simulink model "kalmanHung"  (R2016a)
settings: Solver=VariableStepAuto  StartTime=0.0  StopTime=10  RelTol=1e-3
libraries: commrandsrc3 x1
settings Model: Creator=hung  LastModifiedBy=hung

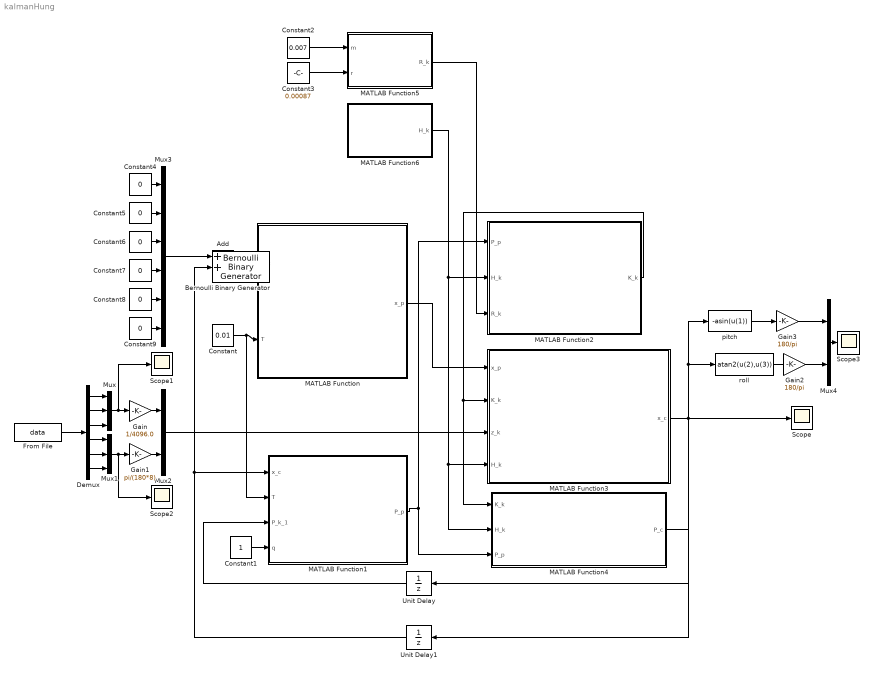
== system kalmanHung ==
  Add : Sum
  Constant : Constant  Value=0.01
  Constant1 : Constant
  Constant2 : Constant  Value=0.007
  Constant3 : Constant  Value=0.00087
  Constant{4..9} (6 alike) : Constant  Value=0
  Demux : Demux  Outputs=6
  From File : FromFile  FileName=data  SampleTime=0.01
  Gain : Gain  Gain=1/4096.0
  Gain1 : Gain  Gain=pi/(180*8)
  Gain2 : Gain  Gain=180/pi
  Gain3 : Gain  Gain=180/pi
  MATLAB Function : MATLAB Function  InitFcn=x_c=[0 0 0 0 0 0 ]'  TreatAsAtomicUnit=on
  MATLAB Function1 : MATLAB Function  TreatAsAtomicUnit=on
  MATLAB Function2 : MATLAB Function  TreatAsAtomicUnit=on
  MATLAB Function3 : MATLAB Function  TreatAsAtomicUnit=on
  MATLAB Function4 : MATLAB Function  TreatAsAtomicUnit=on
  MATLAB Function5 : MATLAB Function  TreatAsAtomicUnit=on
  MATLAB Function6 : MATLAB Function  TreatAsAtomicUnit=on
  Mux : Mux  Inputs=3
  Mux1 : Mux  Inputs=3
  Mux2 : Mux  Inputs=2
  Mux3 : Mux  Inputs=6
  Mux4 : Mux  Inputs=2
  Scope{,1..3} (4 alike) : Scope
  Unit Delay : UnitDelay  InitialCondition=eye(6,6)  SampleTime=-1
  Unit Delay1 : UnitDelay  InitialCondition=zeros(6,1)  SampleTime=-1
  pitch : Fcn  Expr=-asin(u(1))
  roll : Fcn  Expr=atan2(u(2),u(3))
  Bernoulli Binary Generator : commrandsrc3/Bernoulli Binary Generator  IOType=siggen  ProbabilityOfZero=0.5  SeedSource=Auto  Seed=0  SampleTime=1  SamplesPerFrame=1  OutputDataType=double  SimulateUsing=Interpreted execution
  wires:
  MATLAB Function/1(x_p) -> MATLAB Function3/1(x_p)
  MATLAB Function1/1(P_p) -> MATLAB Function4/3(P_p), MATLAB Function2/1(P_p)
  MATLAB Function2/1(K_k) -> MATLAB Function4/1(K_k), MATLAB Function3/2(K_k)
  MATLAB Function4/1(P_c) -> Unit Delay/1
  Constant1/1 -> MATLAB Function1/4(q)
  Constant/1 -> MATLAB Function1/2(T), MATLAB Function/2(T)
  MATLAB Function5/1(R_k) -> MATLAB Function2/3(R_k)
  MATLAB Function6/1(H_k) -> MATLAB Function3/4(H_k), MATLAB Function4/2(H_k), MATLAB Function2/2(H_k)
  Constant2/1 -> MATLAB Function5/1(m)
  Constant3/1 -> MATLAB Function5/2(r)
  From File/1 -> Demux/1
  Demux/1 -> Mux/1
  Demux/2 -> Mux/2
  Demux/3 -> Mux/3
  Demux/4 -> Mux1/1
  Demux/5 -> Mux1/2
  Demux/6 -> Mux1/3
  Mux/1 -> Scope1/1, Gain/1
  Mux1/1 -> Scope2/1, Gain1/1
  Gain/1 -> Mux2/1
  Gain1/1 -> Mux2/2
  Mux2/1 -> MATLAB Function3/3(z_k)
  Add/1 -> MATLAB Function/1(x_c)
  Mux3/1 -> Add/1
  Constant4/1 -> Mux3/1
  Constant5/1 -> Mux3/2
  Constant6/1 -> Mux3/3
  Constant7/1 -> Mux3/4
  Constant8/1 -> Mux3/5
  Constant9/1 -> Mux3/6
  Unit Delay/1 -> MATLAB Function1/3(P_k_1)
  Unit Delay1/1 -> Add/2, MATLAB Function1/1(x_c)
  MATLAB Function3/1(x_c) -> Scope/1, Unit Delay1/1, roll/1, pitch/1
  roll/1 -> Mux4/2
  pitch/1 -> Gain3/1
  Mux4/1 -> Scope3/1
  Gain3/1 -> Mux4/1

== matlab function kalmanHung/MATLAB Function1 ==
  data: x_c input; P_p output; T input; P_k_1 input; q input
function P_p=Predict_P(x_c,T,P_k_1,q)% x_p: x predicted, x_c: x_corrected
C3=[0,-x_c(3),x_c(2);x_c(3),0,-x_c(1);-x_c(2),x_c(1),0];
Ak=[eye(3,3),T*C3;zeros(3,3),eye(3,3)];
Qk=q*[T^3*C3*C3',T^2*C3;T^2*C3',T*eye(3,3)];
P_p=Ak*P_k_1*Ak'+Qk;
end

== matlab function kalmanHung/MATLAB Function ==
  data: x_c input; x_p output; T input
function x_p=Predict_x(x_c,T)% x_p: x predicted, x_c: x_corrected
C3=[0,-x_c(3),x_c(2);x_c(3),0,-x_c(1);-x_c(2),x_c(1),0];
Ak=[eye(3,3),T*C3;zeros(3,3),eye(3,3)];
x_p=Ak*x_c;
end

== matlab function kalmanHung/MATLAB Function2 ==
  data: P_p input; K_k output; H_k input; R_k input
function K_k=K_gain(P_p,H_k,R_k)
K_k=P_p*H_k'*(H_k*P_p*H_k'+R_k);
end

== matlab function kalmanHung/MATLAB Function3 ==
  data: x_p input; K_k input; z_k input; H_k input; x_c output
function x_c=Correct_x(x_p,K_k,z_k,H_k)
x_c=x_p+K_k*(z_k-H_k*x_p);
end

== matlab function kalmanHung/MATLAB Function4 ==
  data: K_k input; P_c output; H_k input; P_p input
function P_c= Correct_P(K_k,H_k,P_p)
P_c=(eye(6,6)-K_k*H_k)*P_p;
end

== matlab function kalmanHung/MATLAB Function5 ==
  data: m input; R_k output; r input
function R_k = Create_R(m,r)
%#codegen
R_k=[m*eye(3,3),zeros(3,3);zeros(3,3),r*eye(3,3)];

== matlab function kalmanHung/MATLAB Function6 ==
  data: H_k output
function H_k = Create_H()
%#codegen

H_k=eye(6,6);
